simulink model "pcm"  (R2018a)
settings: Solver=VariableStepAuto  StartTime=0.0  StopTime=10.0  MaxStep=1e-4  RelTol=1e-3
libraries: dspquant2 x2, commchan3 x1, dsparch4 x1, dspsigops x1
settings Model: Creator=Vibha  LastModifiedBy=vivek
settings CodeAppCC: StateflowObjectComments=on
settings SimscapeCC: SimscapeNormalizeSystem=off

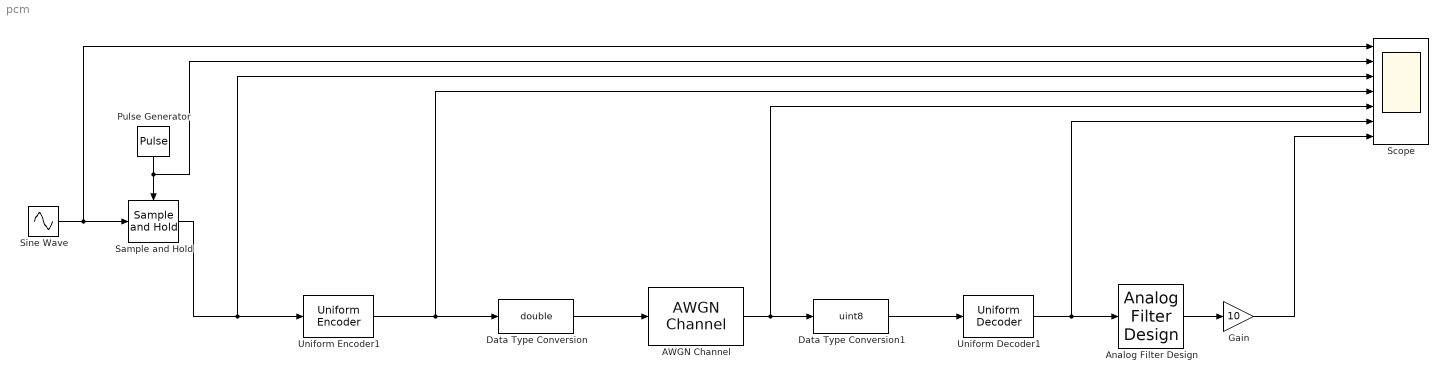
== system pcm ==
  AWGN Channel : commchan3/AWGN Channel  InputProcessing=Columns as channels (frame based)  seed=67  noiseMode="Signal to noise ratio  (SNR)"  EbNodB=10  EsNodB=10  SNRdB=10  bitsPerSym=1  Ps=1  Tsym=0.1  variance=1
  Analog Filter Design : dsparch4/Analog Filter Design  method=Butterworth  filttype=Lowpass  N=8  Wlo=3.5*pi  Whi=3.5*pi  Rp=2  Rs=40
  Data Type Conversion : DataTypeConversion  OutDataTypeStr=double
  Data Type Conversion1 : DataTypeConversion  OutDataTypeStr=uint8
  Gain : Gain  Gain=10
  Pulse Generator : DiscretePulseGenerator  PulseType=Time based  Period=0.1  PulseWidth=5
  Sample and Hold : dspsigops/Sample and Hold  trig=Rising edge  initCond=0  latchinput=off
  Scope : Scope  NumInputPorts=7
  Sine Wave : Sin  Frequency=2*pi  SampleTime=0
  Uniform Decoder1 : dspquant2/Uniform Decoder  peak=1  bits=3  overflowMode=Saturate  otype=Double
      settings: SourceProductName=DSP System Toolbox  SourceProductBaseCode=DS
  Uniform Encoder1 : dspquant2/Uniform Encoder  peak=1  bits=3  otype=Unsigned integer
      settings: SourceProductName=DSP System Toolbox
  wires:
  Analog Filter Design/1 -> Gain/1
  Sine Wave/1 -> Scope/1, Sample and Hold/1
  Pulse Generator/1 -> Scope/2, Sample and Hold/Trigger
  Sample and Hold/1 -> Scope/3, Uniform Encoder1/1
  AWGN Channel/1 -> Scope/5, Data Type Conversion1/1
  Uniform Decoder1/1 -> Scope/6, Analog Filter Design/1
  Uniform Encoder1/1 -> Scope/4, Data Type Conversion/1
  Data Type Conversion1/1 -> Uniform Decoder1/1
  Data Type Conversion/1 -> AWGN Channel/1
  Gain/1 -> Scope/7
